simulink model "lab5"  (R2023a)
settings: Solver=ode45  StartTime=0.0  StopTime=150  MaxStep=0.05  RelTol=1e-3
libraries: simulink x2
settings Model: Creator=bm50345  LastModifiedBy=bm50345

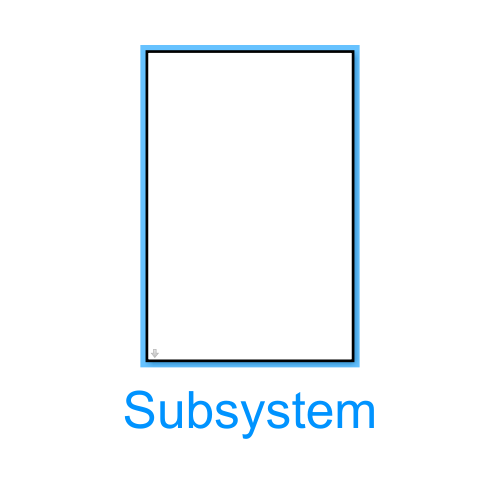
[thumbnail: Simulink's stored preview of the top-level diagram]
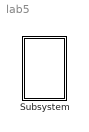
== system lab5 ==
  Subsystem : Subsystem  mask{h1=4, h2=2, S1=1, S2=2, Swy1=0.2, Swy2=0.2, fi1=1, fi2=1, Qwe=2, g=9.81}

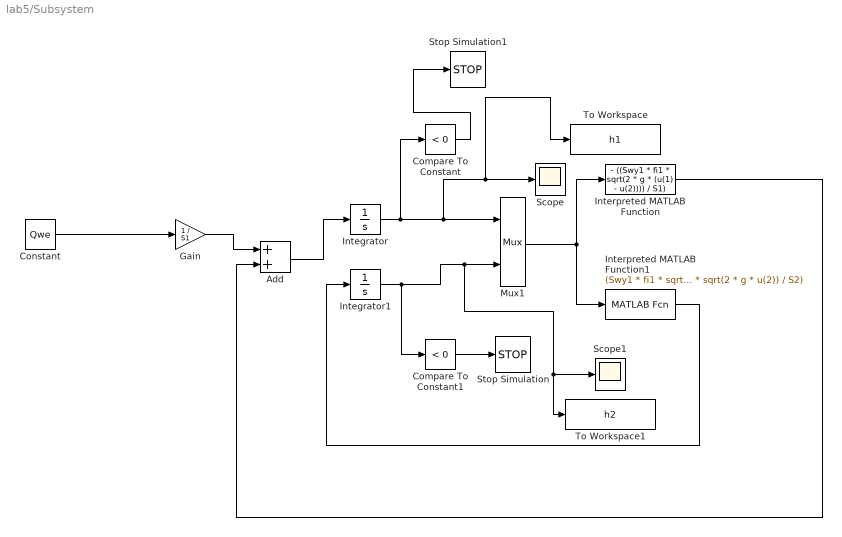
== system lab5/Subsystem ==
  Add : Sum
  Compare To Constant : simulink/Logic and Bit Operations/Compare To Constant  relop=<  const=0  OutDataTypeStr=boolean
  Compare To Constant1 : simulink/Logic and Bit Operations/Compare To Constant  relop=<  const=0  OutDataTypeStr=boolean
  Constant : Constant  Value=Qwe
  Gain : Gain  Gain=1 / S1
  Integrator : Integrator  InitialCondition=h1
  Integrator1 : Integrator  InitialCondition=h2
  Interpreted MATLAB Function : MATLABFcn  MATLABFcn=- ((Swy1 * fi1 * sqrt(2 * g * (u(1) - u(2)))) / S1)
  Interpreted MATLAB Function1 : MATLABFcn  MATLABFcn=(Swy1 * fi1 * sqrt(2 * g * (u(1) - u(2))) / S2) - (Swy2 * fi2 * sqrt(2 * g * u(2)) / S2)
  Mux1 : Mux  Inputs=2
  Scope : Scope
  Scope1 : Scope
  Stop Simulation : Stop
  Stop Simulation1 : Stop
  To Workspace : ToWorkspace  VariableName=h1  SampleTime=-1
  To Workspace1 : ToWorkspace  VariableName=h2  SampleTime=-1
  wires:
  Compare To Constant/1 -> Stop Simulation1/1
  Interpreted MATLAB Function1/1 -> Integrator1/1
  Integrator/1 -> Compare To Constant/1, To Workspace/1, Scope/1, Mux1/1
  Constant/1 -> Gain/1
  Add/1 -> Integrator/1
  Mux1/1 -> Interpreted MATLAB Function/1, Interpreted MATLAB Function1/1
  Interpreted MATLAB Function/1 -> Add/2
  Integrator1/1 -> Compare To Constant1/1, To Workspace1/1, Scope1/1, Mux1/2
  Compare To Constant1/1 -> Stop Simulation/1
  Gain/1 -> Add/1
